simulink model "untitled"  (R2026a)
settings: Solver=VariableStepAuto  StopTime=1
values from neighbouring files (symbols this model uses):
  cs = 1500    [quarter_car_parameters.m]    (also in script.m)
  f = v/lambda    [quarter_car_parameters.m]    (also in script.m)
  ks = 15000    [quarter_car_parameters.m]    (also in script.m)
  kt = 150000    [quarter_car_parameters.m]    (also in script.m)
  ms = 300    [quarter_car_parameters.m]    (also in script.m)
  mu = 40    [quarter_car_parameters.m]    (also in script.m)
settings Model: Creator=ASUS  LastModifiedBy=ASUS

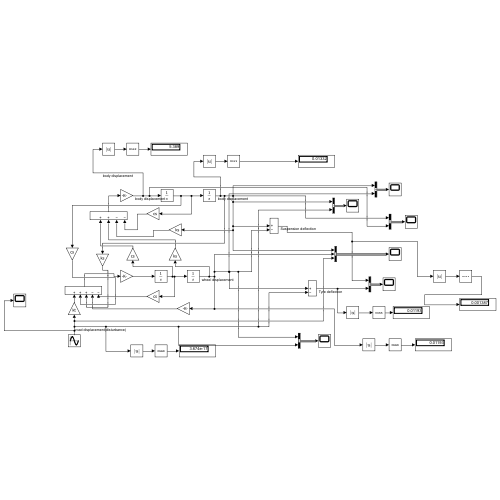
[thumbnail: Simulink's stored preview of the top-level diagram]
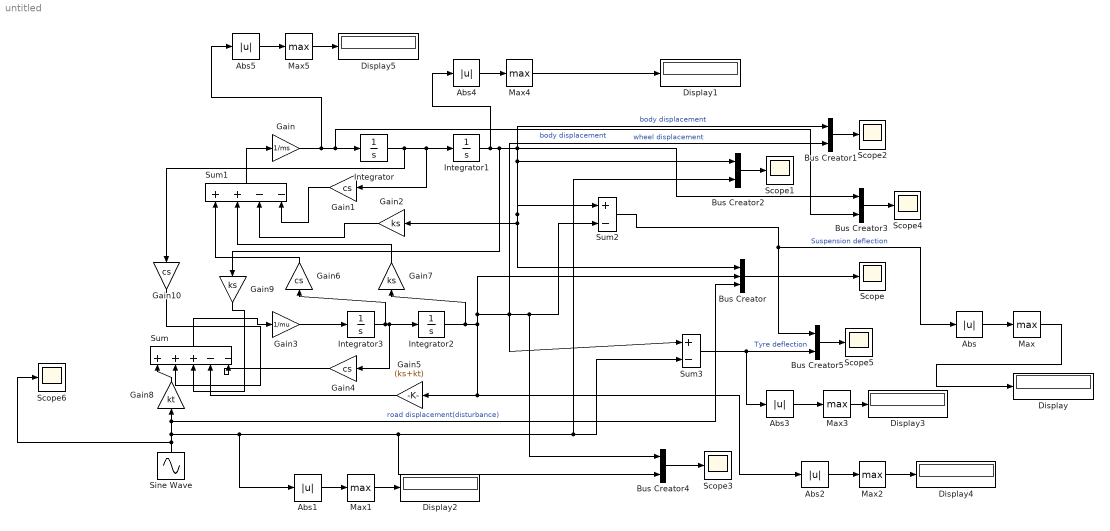
== system untitled ==
  Abs{,1..5} (6 alike) : Abs  SaturateOnIntegerOverflow=off
  Bus Creator : BusCreator  Inputs=3
  Bus Creator{1..5} (5 alike) : BusCreator  Inputs=2
  Display{,1..5} (6 alike) : Display
  Gain : Gain  Gain=1/ms
  Gain{1,4,6,10} (4 alike) : Gain  Gain=cs
  Gain2 : Gain  Gain=ks
  Gain3 : Gain  Gain=1/mu
  Gain5 : Gain  Gain=(ks+kt)
  Gain7 : Gain  Gain=ks
  Gain8 : Gain  Gain=kt
  Gain9 : Gain  Gain=ks
  Integrator{,1..3} (4 alike) : Integrator
  Max{,1..5} (6 alike) : MinMax  Function=max
  Scope{,1..6} (7 alike) : Scope
      Scope settings: ActiveDisplayYMinimum=-0.14807952766653446  ActiveDisplayYMaximum=0.096408110464009059
      Scope1 settings: ActiveDisplayYMinimum=-0.14807952766653446  ActiveDisplayYMaximum=0.096408110464009059
      Scope2 settings: ActiveDisplayYMinimum=-0.14807952766653446  ActiveDisplayYMaximum=0.096408110464009059  DataLoggingVariableName=ScopeData2
      Scope3 settings: ActiveDisplayYMinimum=-0.066465376764334769  ActiveDisplayYMaximum=0.063684073387526519  DataLoggingVariableName=ScopeData3
      Scope4 settings: ActiveDisplayYMinimum=-8.0000084548996888  ActiveDisplayYMaximum=7.9123529077769064  DataLoggingVariableName=ScopeData4
      Scope5 settings: ActiveDisplayYMinimum=-0.12286295236262358  ActiveDisplayYMaximum=0.085720122897160633  DataLoggingVariableName=ScopeData5
      Scope6 settings: ActiveDisplayYMinimum=-1  ActiveDisplayYMaximum=1  DataLoggingVariableName=ScopeData6
  Sine Wave : Sin  Amplitude=0.05  Frequency=2*pi*f  SampleTime=0
  Sum : Sum  Inputs=|+++--
  Sum1 : Sum  Inputs=|++--
  Sum2 : Sum  Inputs=|+-
  Sum3 : Sum  Inputs=|+-
  wires:
  Integrator/1 -> Gain10/1, Gain1/1, Integrator1/1
  Integrator1/1 -> Abs4/1, Bus Creator3/1, Bus Creator/1, Gain2/1, Sum2/1, Bus Creator2/1, Bus Creator1/1, Gain9/1  "body displacement"
  Gain3/1 -> Integrator3/1
  Integrator3/1 -> Gain6/1, Gain4/1, Integrator2/1
  Integrator2/1 -> Abs2/1, Gain5/1, Bus Creator1/2, Sum3/1, Bus Creator4/1, Sum2/2, Bus Creator/2, Gain7/1  "wheel displacement"
  Gain10/1 -> Sum/2
  Gain9/1 -> Sum/3
  Sum/1 -> Gain3/1
  Gain4/1 -> Sum/5
  Gain5/1 -> Sum/4
  Gain1/1 -> Sum1/4
  Gain2/1 -> Sum1/3
  Gain6/1 -> Sum1/1
  Gain7/1 -> Sum1/2
  Sum1/1 -> Gain/1
  Gain8/1 -> Sum/1
  Sine Wave/1 -> Scope6/1, Abs1/1, Bus Creator4/2, Bus Creator2/2, Sum3/2, Bus Creator/3, Gain8/1  "road displacement(disturbance)"
  Bus Creator/1 -> Scope/1
  Sum2/1 -> Abs/1, Bus Creator5/1  "Suspension deflection"
  Sum3/1 -> Abs3/1, Bus Creator5/2  "Tyre deflection"
  Bus Creator4/1 -> Scope3/1
  Bus Creator2/1 -> Scope1/1
  Bus Creator1/1 -> Scope2/1
  Bus Creator3/1 -> Scope4/1
  Bus Creator5/1 -> Scope5/1
  Abs/1 -> Max/1
  Max/1 -> Display/1
  Abs4/1 -> Max4/1
  Max4/1 -> Display1/1
  Abs3/1 -> Max3/1
  Abs2/1 -> Max2/1
  Abs1/1 -> Max1/1
  Max2/1 -> Display4/1
  Max3/1 -> Display3/1
  Max1/1 -> Display2/1
  Gain/1 -> Abs5/1, Bus Creator3/2, Integrator/1  "body displacement"
  Max5/1 -> Display5/1
  Abs5/1 -> Max5/1
